simulink model "DSM_discrete"  (Simulink 7.8)
settings: Solver=FixedStepDiscrete  StartTime=0.0  StopTime=inf  FixedStep=Delta_t  RelTol=1e-3
undefined symbols (not defined in the file or in its folder): Delta_t, q
settings Model: Creator=imac  LastModifiedBy=aitor
settings DebuggingCC: FcnCallInpInsideContextMsg=Use local settings

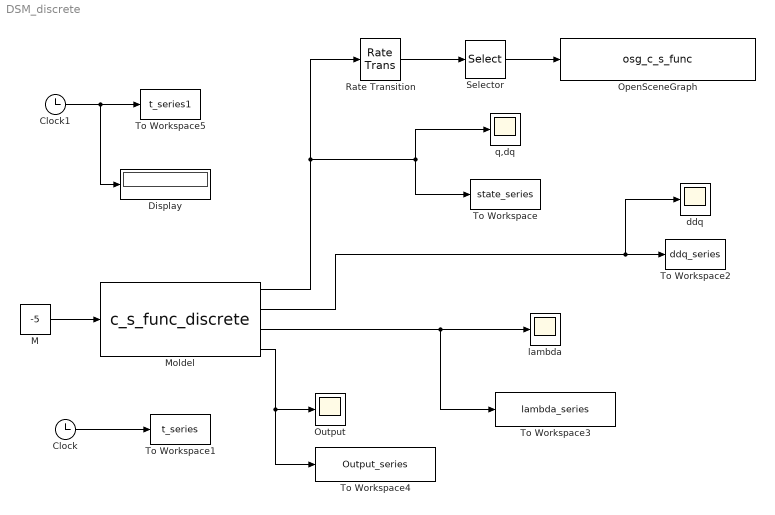
== system DSM_discrete ==
  Clock : Clock
  Clock1 : Clock
  Display : Display
  M : Constant  Value=-5  SampleTime=Delta_t
  Moldel : S-Function  FunctionName=c_s_func_discrete  Parameters=q dq param Delta_t  EnableBusSupport=off
      mask Type: S-function: mycsfunc
      mask Description: This is a S-function that does the continuous state space system.
      mask Display: disp('[M , Phi_q''] [ddq]\n[Phi_q , 0] [lambda]\n=\n [Q ] \n   [gamma] ');
  OpenSceneGraph : S-Function  FunctionName=osg_c_s_func  EnableBusSupport=off
  Output : Scope
      settings: YMin=-1750  YMax=1000  SaveName=ScopeData3  SampleInput=on
  Rate Transition : RateTransition  OutPortSampleTime=0.04
  Selector : Selector  InputPortWidth=2*length(q)  IndexOptions=Index vector (dialog)  Indices=1:1:length(q)  OutputSizes=1
  To Workspace : ToWorkspace  VariableName=state_series  SampleTime=-1  SaveFormat=Array
  To Workspace1 : ToWorkspace  VariableName=t_series  SampleTime=-1  SaveFormat=Array
  To Workspace2 : ToWorkspace  VariableName=ddq_series  SampleTime=-1  SaveFormat=Array
  To Workspace3 : ToWorkspace  VariableName=lambda_series  SampleTime=-1  SaveFormat=Array
  To Workspace4 : ToWorkspace  VariableName=Output_series  SampleTime=-1  SaveFormat=Array
  To Workspace5 : ToWorkspace  VariableName=t_series1  SampleTime=Delta_t  SaveFormat=Array
  ddq : Scope
      settings: YMin=-500  YMax=300  SampleInput=on
  lambda : Scope
      settings: YMin=-1750  YMax=1000  SaveName=ScopeData2  SampleInput=on
  q,dq : Scope
      settings: YMin=-15  YMax=15  SampleInput=on
  wires:
  Clock/1 -> To Workspace1/1
  Moldel/1 -> q,dq/1, To Workspace/1, Rate Transition/1
  Moldel/2 -> ddq/1, To Workspace2/1
  Moldel/3 -> lambda/1, To Workspace3/1
  M/1 -> Moldel/1
  Selector/1 -> OpenSceneGraph/1
  Rate Transition/1 -> Selector/1
  Moldel/4 -> To Workspace4/1, Output/1
  Clock1/1 -> Display/1, To Workspace5/1
